simulink model "Simple_LMS"  (R2014b)
settings: Solver=ode45  StartTime=0.0  StopTime=5000  RelTol=1e-3
values from neighbouring files (symbols this model uses):
  vref = 0.75    [DFE_LMS_example.m]
libraries: simulink x5, ams_primitives x1
settings Model: Creator=Jase  LastModifiedBy=Jase

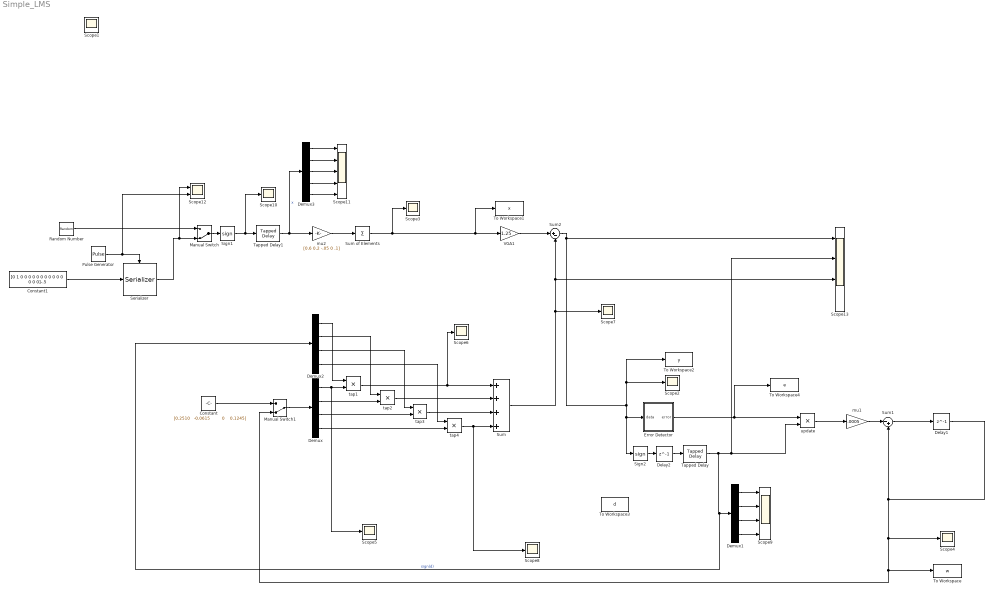
== system Simple_LMS ==
  Constant : Constant  Value="[0.2510   -0.0615         0    0.1245]"
  Constant1 : Constant  Value=[0 1 0 0 0 0 0 0 0 0 0 0 0 0 0 0]-.5
  Delay1 : Delay  DelayLength=1  InitialCondition=0.1  SampleTime=1
  Delay2 : Delay  DelayLength=1  InitialCondition=0.1
  Demux : Demux
  Demux1 : Demux
  Demux2 : Demux
  Demux3 : Demux  Outputs=5
  Error Detector : Subsystem
  Manual Switch : ManualSwitch  CurrentSetting=0
  Manual Switch1 : ManualSwitch  CurrentSetting=0
  Pulse Generator : DiscretePulseGenerator  PulseType=Time based  Period=1  PulseWidth=50
  Random Number : RandomNumber  SampleTime=1
  Scope{1..8,10} (9 alike) : Scope
      Scope10 settings: ShowLegends=on  YMin=0.2  YMax=1.2  SaveName=ScopeData11
      Scope2 settings: ShowLegends=on  YMin=0.1  YMax=0.9
      Scope3 settings: ShowLegends=on  YMin=0.2  YMax=1.2  SaveName=ScopeData2
      Scope4 settings: ShowLegends=on  SaveName=ScopeData5
      Scope5 settings: ShowLegends=on  SaveName=ScopeData7
      Scope6 settings: ShowLegends=on  SaveName=ScopeData8
      Scope7 settings: ShowLegends=on  SaveName=ScopeData9
      Scope8 settings: ShowLegends=on  SaveName=ScopeData10
      Scope1 settings: SaveName=ScopeData6
  Scope11 : Scope  NumInputPorts=5
      settings: ShowLegends=on  YMin=0.2~-5~-5~-5~-5  YMax=1.2~5~5~5~5  SaveName=ScopeData12
  Scope12 : Scope  NumInputPorts=2
      settings: ShowLegends=on  YMin=0.2~-5  YMax=1.2~5  SaveName=ScopeData13
  Scope13 : Scope  NumInputPorts=4
      settings: ShowLegends=on  YMin=-5~-5~-5~-5  YMax=5~5~5~5  SaveName=ScopeData14
  Scope9 : Scope  NumInputPorts=4
      settings: ShowLegends=on  YMin=0.1~-5~-5~-5  YMax=0.9~5~5~5  SaveName=ScopeData3
  Serializer : ams_primitives/Serializer  N=16
  Sign1 : Signum  SampleTime=1
  Sign2 : Signum
  Sum : Sum  Inputs=++++
  Sum of Elements : Sum  Inputs=+
  Sum1 : Sum  Inputs=|-+  OutDataTypeStr=double
  Sum2 : Sum  Inputs=|+-  OutDataTypeStr=double
  Tapped Delay : simulink/Discrete/Tapped Delay  vinit=0.0  samptime=-1  NumDelays=3  DelayOrder=Newest  includeCurrent=on
  Tapped Delay1 : simulink/Discrete/Tapped Delay  vinit=0.0  samptime=-1  NumDelays=4  DelayOrder=Newest  includeCurrent=on
  To Workspace : ToWorkspace  VariableName=w  SampleTime=-1
  To Workspace1 : ToWorkspace  VariableName=x  SampleTime=-1
  To Workspace2 : ToWorkspace  VariableName=y  SampleTime=-1
  To Workspace3 : ToWorkspace  VariableName=d  SampleTime=-1
  To Workspace4 : ToWorkspace  VariableName=e  SampleTime=-1
  VGA1 : Gain  Gain=1.25
  mu1 : Gain  Gain=.0005
  mu2 : Gain  Gain=[0.6 0.2 -.05 0 .1]
  tap{1..4} (4 alike) : Product
  update : Product
  wires:
  Demux2/4 -> tap4/1
  Demux2/3 -> tap3/1
  Demux2/2 -> tap2/1
  Demux2/1 -> tap1/1
  Tapped Delay1/1 -> Demux3/1, mu2/1  "x"
  tap2/1 -> Sum/2
  Demux/4 -> tap4/2
  Demux/2 -> tap2/2
  Demux/3 -> tap3/2
  Demux/1 -> Scope5/1, tap1/2
  tap3/1 -> Sum/3
  tap1/1 -> Scope6/1, Sum/1
  tap4/1 -> Scope8/1, Sum/4
  Tapped Delay/1 -> Demux2/1, Demux1/1, Scope13/2, update/2  "sign(d)"
  Sum2/1 -> Scope13/1, Scope2/1, To Workspace2/1, Sign2/1, Error Detector/1(data)
  Sum1/1 -> Delay1/1
  update/1 -> mu1/1
  mu1/1 -> Sum1/1
  Error Detector/1(error) -> To Workspace4/1, update/1
  mu2/1 -> Sum of Elements/1
  Sign1/1 -> Scope10/1, Tapped Delay1/1
  Sum of Elements/1 -> Scope3/1, VGA1/1, To Workspace1/1
  VGA1/1 -> Sum2/1
  Sum/1 -> Scope7/1, Sum2/2, Scope13/3
  Sign2/1 -> Delay2/1
  Demux1/1 -> Scope9/1
  Demux1/2 -> Scope9/2
  Demux1/3 -> Scope9/3
  Demux1/4 -> Scope9/4
  Delay2/1 -> Tapped Delay/1
  Pulse Generator/1 -> Scope12/2, Serializer/Trigger
  Manual Switch/1 -> Sign1/1
  Random Number/1 -> Manual Switch/1
  Serializer/1 -> Scope12/1, Manual Switch/2
  Constant1/1 -> Serializer/1
  Demux3/1 -> Scope11/1
  Demux3/2 -> Scope11/2
  Demux3/3 -> Scope11/3
  Demux3/4 -> Scope11/4
  Demux3/5 -> Scope11/5
  Manual Switch1/1 -> Demux/1
  Delay1/1 -> Scope4/1, Manual Switch1/2, To Workspace/1, Sum1/2
  Constant/1 -> Manual Switch1/1

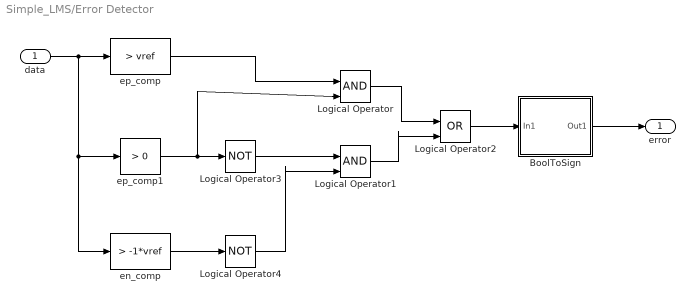
== system Simple_LMS/Error Detector ==
  data : Inport
  BoolToSign : Subsystem
  Logical Operator : Logic  IconShape=distinctive  AllPortsSameDT=off  OutDataTypeStr=boolean
  Logical Operator1 : Logic  IconShape=distinctive  AllPortsSameDT=off  OutDataTypeStr=boolean
  Logical Operator2 : Logic  Operator=OR  IconShape=distinctive  AllPortsSameDT=off  OutDataTypeStr=boolean
  Logical Operator3 : Logic  Operator=NOT  IconShape=distinctive  AllPortsSameDT=off  OutDataTypeStr=boolean
  Logical Operator4 : Logic  Operator=NOT  IconShape=distinctive  AllPortsSameDT=off  OutDataTypeStr=boolean
  en_comp : simulink/Logic and Bit Operations/Compare To Constant  relop=>  const=-1*vref  OutDataTypeStr=uint8
  ep_comp : simulink/Logic and Bit Operations/Compare To Constant  relop=>  const=vref  OutDataTypeStr=uint8
  ep_comp1 : simulink/Logic and Bit Operations/Compare To Constant  relop=>  const=0  OutDataTypeStr=uint8
  error : Outport
  wires:
  Logical Operator/1 -> Logical Operator2/1
  Logical Operator2/1 -> BoolToSign/1(In1)
  Logical Operator1/1 -> Logical Operator2/2
  Logical Operator3/1 -> Logical Operator1/1
  ep_comp1/1 -> Logical Operator/2, Logical Operator3/1
  data/1 -> en_comp/1, ep_comp1/1, ep_comp/1
  ep_comp/1 -> Logical Operator/1
  BoolToSign/1(Out1) -> error/1
  Logical Operator4/1 -> Logical Operator1/2
  en_comp/1 -> Logical Operator4/1

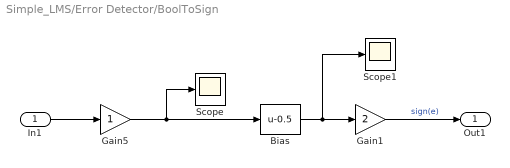
== system Simple_LMS/Error Detector/BoolToSign ==
  In1 : Inport
  Bias : Bias  Bias=-0.5
  Gain1 : Gain  Gain=2
  Gain5 : Gain  OutDataTypeStr=double
  Scope : Scope
  Scope1 : Scope
      settings: SaveName=ScopeData4
  Out1 : Outport
  wires:
  Bias/1 -> Scope1/1, Gain1/1
  Gain1/1 -> Out1/1  "sign(e)"
  In1/1 -> Gain5/1
  Gain5/1 -> Scope/1, Bias/1
